simulink model "vrtut3"  (Simulink 7.4)
settings: Solver=ode45  StartTime=0.0  StopTime=Inf  RelTol=1e-3
libraries: vrlib x2
Description:
  | Simulink(R) 3D Animation(TM) - Tutorial #3
  | 
  | Tutorial model to be used for V-Realm authoring example in the User's manual.
  | After creating the virtual world according to the instructions in the manual, include the VR block
  | in the model and connect B1, B2 coordinates and S scaling to corresponding nodes in
  | the virtual world.
settings Model: Creator=Danek  LastModifiedBy=Houska  CovMetricSettings=d  ExtModeTrigMode=oneshot  ExtModeArmWhenConnect=off
settings DataIOCC: SaveOutput=off  SaveTime=off  SignalLoggingName=logsOut
settings OptimizationCC: BooleanDataType=off  InlineInvariantSignals=on  InitFltsAndDblsToZero=on
settings DebuggingCC: CheckExecutionContextPreStartOutputMsg=on  CheckExecutionContextRuntimeOutputMsg=on  SignalResolutionControl=TryResolveAllWithWarning  SolverPrmCheckMsg=none  MultiTaskDSMMsg=warning  MultiTaskCondExecSysMsg=none  StrictBusMsg=None
settings HardwareCC: TargetUnknown=on
settings ModelReferenceCC: UpdateModelReferenceTargets=IfOutOfDate
settings SFSimCC: SimGenerateEmlReport=off
settings RTWCC: IncludeERTFirstTime=on
settings GRTTargetCC: TargetFcnLib=ansi_tfl_tmw.mat

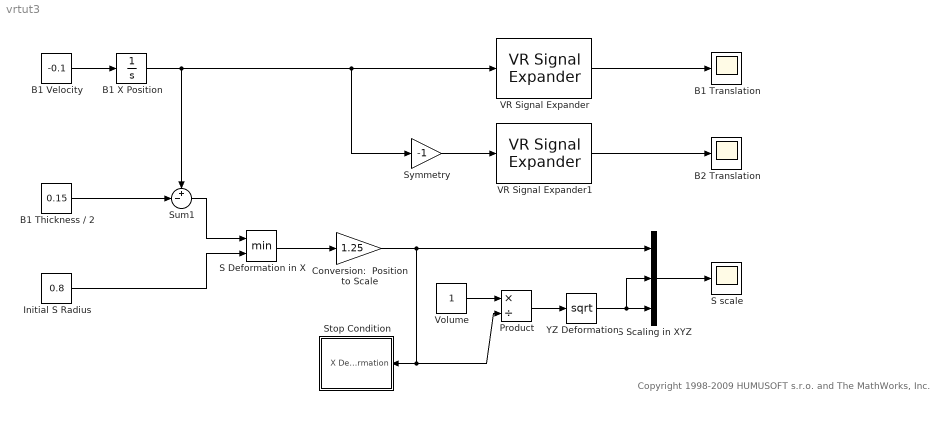
== system vrtut3 ==
  note: Copyright 1998-2009 HUMUSOFT s.r.o. and The MathWorks, Inc.
  B1 Thickness / 2 : Constant  Value=0.15  OutDataType=sfix(16)  OutScaling=2^0
  B1 Translation : Scope
  B1 Velocity : Constant  Value=-0.1  OutDataType=sfix(16)  OutScaling=2^0
  B1 X Position : Integrator  InitialCondition=3  UpperSaturationLimit=Inf  LowerSaturationLimit=-Inf
  B2 Translation : Scope
  Conversion:  Position to Scale : Gain  Gain=1.25  ParameterDataType=sfix(16)  ParameterScaling=2^0  OutDataType=sfix(16)  OutScaling=2^0  SaturateOnIntegerOverflow=on  OutDataTypeStr=Inherit: Same as input  ParamDataTypeStr=Inherit: Same as input
  Initial S Radius : Constant  Value=0.8  OutDataType=sfix(16)  OutScaling=2^0
  Product : Product  Inputs=*/  OutDataType=sfix(16)  OutScaling=2^0  SaturateOnIntegerOverflow=on  RndMeth=Zero  InputSameDT=on  OutDataTypeStr=Inherit: Same as first input
  "S Deformation in X " : MinMax  Inputs=2  OutDataType=sfix(16)  OutScaling=2^0  SaturateOnIntegerOverflow=on  InputSameDT=on
  S Scaling in XYZ : Mux  Inputs=3
  S scale : Scope
  Stop Condition : Subsystem
  Sum1 : Sum  Inputs=+-|  OutDataType=sfix(16)  OutScaling=2^0  SaturateOnIntegerOverflow=on  InputSameDT=on  OutDataTypeStr=Inherit: Same as first input
  Symmetry : Gain  Gain=-1  ParameterDataType=sfix(16)  ParameterScaling=2^0  OutDataType=sfix(16)  OutScaling=2^0  SaturateOnIntegerOverflow=on  OutDataTypeStr=Inherit: Same as input  ParamDataTypeStr=Inherit: Same as input
  VR Signal Expander : vrlib/VR Signal Expander  SystemSampleTime=-1  outwidth=3  outidx=1
  VR Signal Expander1 : vrlib/VR Signal Expander  SystemSampleTime=-1  outwidth=3  outidx=1
  Volume : Constant  OutDataType=sfix(16)  OutScaling=2^0
  YZ Deformation : Math  Operator=sqrt  OutDataType=sfix(16)  OutScaling=2^0  SaturateOnIntegerOverflow=on
  wires:
  Symmetry/1 -> VR Signal Expander1/1
  B1 X Position/1 -> Symmetry/1, VR Signal Expander/1, Sum1/1
  "S Deformation in X "/1 -> Conversion:  Position to Scale/1
  B1 Velocity/1 -> B1 X Position/1
  B1 Thickness / 2/1 -> Sum1/2
  Initial S Radius/1 -> "S Deformation in X "/2
  Sum1/1 -> "S Deformation in X "/1
  Conversion:  Position to Scale/1 -> Product/2, Stop Condition/1(X Deformation), S Scaling in XYZ/1
  Volume/1 -> Product/1
  Product/1 -> YZ Deformation/1
  YZ Deformation/1 -> S Scaling in XYZ/2, S Scaling in XYZ/3
  S Scaling in XYZ/1 -> S scale/1
  VR Signal Expander/1 -> B1 Translation/1
  VR Signal Expander1/1 -> B2 Translation/1

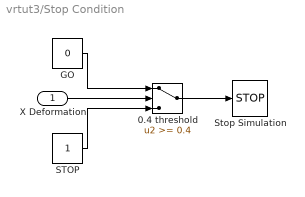
== system vrtut3/Stop Condition ==
  X Deformation : Inport  OutDataType=sfix(16)  OutScaling=2^0
  0.4 threshold : Switch  Threshold=0.4  OutDataType=sfix(16)  OutScaling=2^0  SaturateOnIntegerOverflow=on  InputSameDT=on
  GO : Constant  Value=0  OutDataType=sfix(16)  OutScaling=2^0
  STOP : Constant  OutDataType=sfix(16)  OutScaling=2^0
  Stop Simulation : Stop
  wires:
  X Deformation/1 -> 0.4 threshold/2
  GO/1 -> 0.4 threshold/1
  STOP/1 -> 0.4 threshold/3
  0.4 threshold/1 -> Stop Simulation/1
